simulink model "fuzzy1_MATLAB_2012b"  (Simulink 8.0)
settings: Solver=ode3  StartTime=0.0  StopTime=1  FixedStep=0.001  RelTol=1e-3
libraries: fuzblock x1
settings Model: Creator=yulong  ModifiedByFormat=我爱技术宅  LastModifiedBy=我爱技术宅
settings SolverCC: ZeroCrossControl=DisableAll
settings DataIOCC: SignalLoggingSaveFormat=ModelDataLogs
settings OptimizationCC: ExpressionDepthLimit=128  InitFltsAndDblsToZero=on
settings DebuggingCC: SaveWithParameterizedLinksMsg=none  SignalResolutionControl=TryResolveAllWithWarning  MultiTaskDSMMsg=warning  MultiTaskCondExecSysMsg=none  FcnCallInpInsideContextMsg=EnableAllAsWarning  FrameProcessingCompatibilityMsg=error  StateNameClashWarn=none
settings CodeAppCC: CustomSymbolStrType=$N$R$M_T
settings GRTTargetCC: TargetFcnLib=ansi_tfl_tmw.mat  CodeReplacementLibrary=C89/C90 (ANSI)  GeneratePreprocessorConditionals=Use local settings  CombineOutputUpdateFcns=off  GRTInterface=on

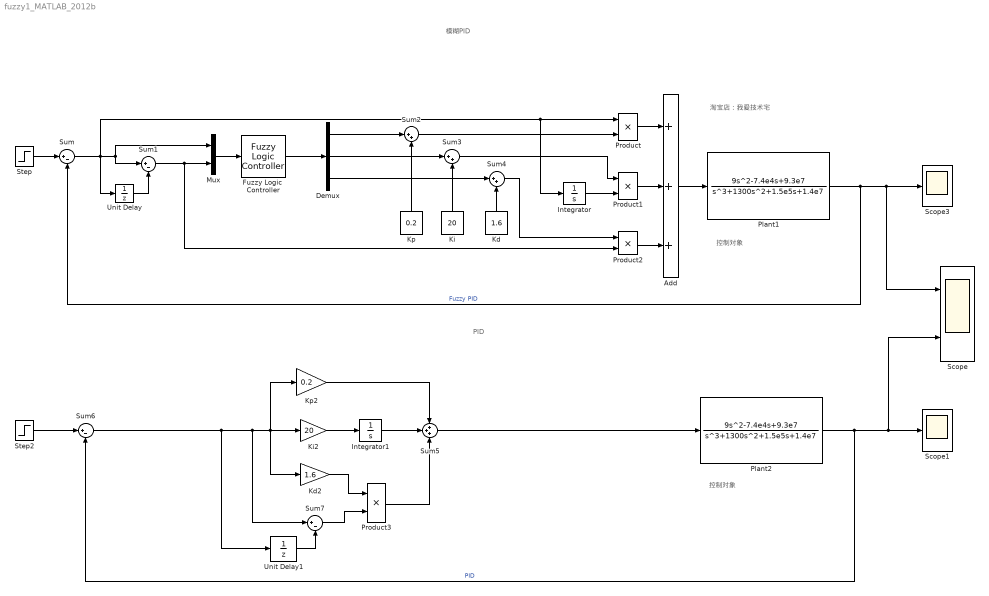
== system fuzzy1_MATLAB_2012b ==
  note: 控制对象
  note: 淘宝店：我爱技术宅
  note: 模糊PID
  note: 控制对象
  note: PID
  Add : Sum  Inputs=3
  Demux : Demux  Outputs=3
  Fuzzy Logic  Controller : fuzblock/Fuzzy Logic  Controller  FIS='fuzzypid.fis'
  Integrator : Integrator
  Integrator1 : Integrator
  Kd : Constant  Value=1.6
  Kd2 : Gain  Gain=1.6
  Ki : Constant  Value=20
  Ki2 : Gain  Gain=20
  Kp : Constant  Value=0.2
  Kp2 : Gain  Gain=0.2
  Mux : Mux  Inputs=2
  Plant1 : TransferFcn  Numerator=[9 -7.4e4 9.3e7]  Denominator=[1 1300 1.5e5 1.4e7]
  Plant2 : TransferFcn  Numerator=[9 -7.4e4 9.3e7]  Denominator=[1 1300 1.5e5 1.4e7]
  Product : Product
  Product1 : Product
  Product2 : Product
  Product3 : Product  RndMeth=Zero
  Scope : Scope  NumInputPorts=2
      settings: TimeRange=auto  ShowLegends=on  MaxDataPoints=5000  SaveToWorkspace=off  SaveName=ScopeData  YMin=-0.13976~-5  YMax=1.25785~5  SampleTime=-1
  Scope1 : Scope
      settings: TimeRange=auto  ShowLegends=on  MaxDataPoints=5000  SaveToWorkspace=off  YMin=-0.13976  YMax=1.25785  SampleTime=-1
  Scope3 : Scope
      settings: TimeRange=auto  ShowLegends=on  MaxDataPoints=5000  SaveToWorkspace=off  SaveName=ScopeData3  YMin=-0.13366  YMax=1.20298  SampleTime=-1
  Step : Step  Time=0  SampleTime=0
  Step2 : Step  Time=0  SampleTime=0
  Sum{,1,6..7} (4 alike) : Sum  Inputs=|+-
  Sum2 : Sum  Inputs=|++
  Sum3 : Sum  Inputs=|++
  Sum4 : Sum  Inputs=|++
  Sum5 : Sum  Inputs=+++
  Unit Delay : UnitDelay  SampleTime=-1  HasFrameUpgradeWarning=on
  Unit Delay1 : UnitDelay  SampleTime=-1  HasFrameUpgradeWarning=on
  wires:
  Step/1 -> Sum/1
  Sum/1 -> Product/1, Integrator/1, Unit Delay/1, Mux/1, Sum1/1
  Mux/1 -> Fuzzy Logic  Controller/1
  Unit Delay/1 -> Sum1/2
  Sum1/1 -> Product2/2, Mux/2
  Fuzzy Logic  Controller/1 -> Demux/1
  Demux/1 -> Sum2/1
  Kp/1 -> Sum2/2
  Demux/2 -> Sum3/1
  Ki/1 -> Sum3/2
  Demux/3 -> Sum4/1
  Kd/1 -> Sum4/2
  Sum2/1 -> Product/2
  Sum3/1 -> Product1/1
  Integrator/1 -> Product1/2
  Plant1/1 -> Sum/2, Scope3/1, Scope/1  "Fuzzy PID"
  Sum4/1 -> Product2/1
  Product2/1 -> Add/3
  Product1/1 -> Add/2
  Product/1 -> Add/1
  Add/1 -> Plant1/1
  Kd2/1 -> Product3/1
  Ki2/1 -> Integrator1/1
  Integrator1/1 -> Sum5/2
  Kp2/1 -> Sum5/1
  Sum5/1 -> Plant2/1
  Unit Delay1/1 -> Sum7/2
  Sum6/1 -> Unit Delay1/1, Sum7/1, Kp2/1, Kd2/1, Ki2/1
  Sum7/1 -> Product3/2
  Product3/1 -> Sum5/3
  Step2/1 -> Sum6/1
  Plant2/1 -> Sum6/2, Scope/2, Scope1/1  "PID"
